simulink model "modelSS"  (R2021b)
settings: Solver=VariableStepAuto  StartTime=0.0  StopTime=100000.0  RelTol=1e-3
undefined symbols (not defined in the file or in its folder): A, B, Bd, C, K, omega_op, T_ambi_op, Theta_1_op, Theta_2_op, U_fan_1_op, U_fan_2_op
settings Model: Creator=martin  LastModifiedBy=kaspe

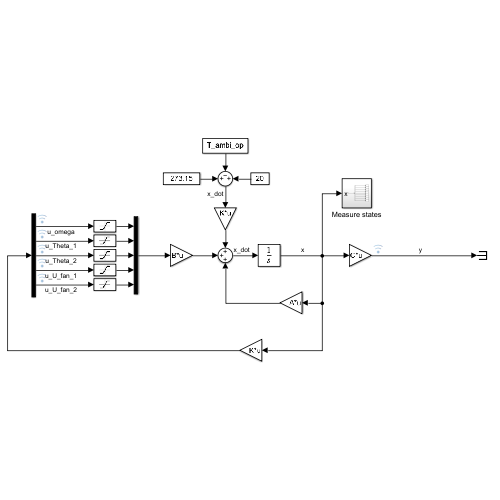
[thumbnail: Simulink's stored preview of the top-level diagram]
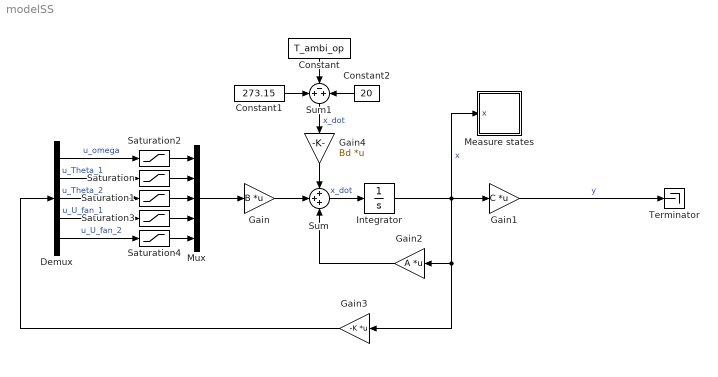
== system modelSS ==
  Constant : Constant  Value=T_ambi_op
  Constant1 : Constant  Value=273.15  VectorParams1D=off
  Constant2 : Constant  Value=20  VectorParams1D=off
  Demux : Demux  Outputs=5
  Gain : Gain  Gain=B  Multiplication=Matrix(K*u)
  Gain1 : Gain  Gain=C  Multiplication=Matrix(K*u)
  Gain2 : Gain  Gain=A  Multiplication=Matrix(K*u)
  Gain3 : Gain  Gain=-K  Multiplication=Matrix(K*u)
  Gain4 : Gain  Gain=Bd  Multiplication=Matrix(K*u)
  Integrator : Integrator  InitialCondition=ones(9,1)
  Measure states : Subsystem
  Mux : Mux  Inputs=5
  Saturation : Saturate  UpperLimit=1-Theta_1_op  LowerLimit=-Theta_1_op
  Saturation1 : Saturate  UpperLimit=1-Theta_2_op  LowerLimit=-Theta_2_op
  Saturation2 : Saturate  UpperLimit=100-omega_op  LowerLimit=-omega_op
  Saturation3 : Saturate  UpperLimit=3600-U_fan_1_op  LowerLimit=-U_fan_1_op
  Saturation4 : Saturate  UpperLimit=3600-U_fan_2_op  LowerLimit=-U_fan_2_op
  Sum : Sum  Inputs=+++
  Sum1 : Sum  Inputs=+-+
  Terminator : Terminator
  wires:
  Sum/1 -> Integrator/1  "x_dot"
  Integrator/1 -> Measure states/1(x), Gain3/1, Gain2/1, Gain1/1  "x"
  Gain2/1 -> Sum/3
  Gain/1 -> Sum/2
  Gain1/1 -> Terminator/1  "y"
  Gain4/1 -> Sum/1
  Sum1/1 -> Gain4/1  "x_dot"
  Constant/1 -> Sum1/2
  Constant1/1 -> Sum1/1
  Saturation1/1 -> Mux/3
  Demux/1 -> Saturation2/1  "u_omega"
  Demux/3 -> Saturation1/1  "u_Theta_2"
  Saturation/1 -> Mux/2
  Gain3/1 -> Demux/1
  Mux/1 -> Gain/1
  Demux/2 -> Saturation/1  "u_Theta_1"
  Demux/5 -> Saturation4/1  "u_U_fan_2"
  Saturation3/1 -> Mux/4
  Saturation4/1 -> Mux/5
  Saturation2/1 -> Mux/1
  Demux/4 -> Saturation3/1  "u_U_fan_1"
  Constant2/1 -> Sum1/3

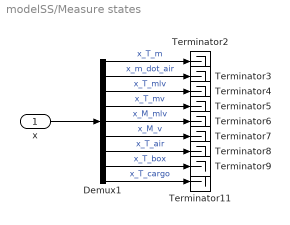
== system modelSS/Measure states ==
  x : Inport
  Demux1 : Demux  Outputs=9
  Terminator{2..9,11} (9 alike) : Terminator
  wires:
  Demux1/5 -> Terminator6/1  "x_M_mlv"
  Demux1/7 -> Terminator8/1  "x_T_air"
  Demux1/6 -> Terminator7/1  "x_M_v"
  Demux1/3 -> Terminator4/1  "x_T_mlv"
  Demux1/1 -> Terminator2/1  "x_T_m"
  Demux1/2 -> Terminator3/1  "x_m_dot_air"
  Demux1/4 -> Terminator5/1  "x_T_mv"
  Demux1/9 -> Terminator11/1  "x_T_cargo"
  Demux1/8 -> Terminator9/1  "x_T_box"
  x/1 -> Demux1/1
